simulink model "DoublePendSim"  (R2022b)
settings: Solver=ode1be  StartTime=0.0  StopTime=3  FixedStep=0.01  RelTol=1e-3
model workspace (MAT data in the model file):
  E = Simulink.Parameter
  E.Value = [1; 1; 0.5; 0; 0.5; 0]
  E.DataType = 'auto'
  E.Complexity = 'real'
  E.Dimensions = [6 1]
  F = Simulink.Parameter
  F.Value = [-1137.64638281  0.333333333333  284.601832874  -0.333333333333  -32.6215233406  -0.333333333333; 1935122.34305  -0.666666666667  -1227588.90432  -0.333333333333  -1810907.99136  -0.333333333333; 314.687310794  -0.333333333333  -490.937143366  0.833333333333  -190.967975417  -0.166666666667; 1036610.18685  0  -658628.221442  0  -949391.226529  0; -27.639193223  -0.333333333333  -190.739049358  -0.166666666667  -1000.74980716  0.833333333333; 1028988.90962  0  -652879.570619  0  -976734.231834  0]
  F.DataType = 'auto'
  F.Complexity = 'real'
  F.Dimensions = [6 6]
  H = Simulink.Parameter
  H.Value = [0.666666666667  0.333333333333  0.333333333333; 0.666666666667  0.333333333333  0.333333333333; 0.333333333333  0.166666666667  0.166666666667; 0  0  0; 0.333333333333  0.166666666667  0.166666666667; 0  0  0]
  H.DataType = 'auto'
  H.Complexity = 'real'
  H.Dimensions = [6 3]
  K1 = Simulink.Parameter
  K1.Value = [1137.64638281  -284.601832874  32.6215233406; -1935122.34305  1227578.3936  1810909.04243; -314.687310794  490.937143366  190.967975417; -1036610.18685  658699.6943  949372.307244; 27.639193223  190.739049358  1000.74980716; -1028988.90962  652728.216333  976843.543262]
  K1.DataType = 'auto'
  K1.Complexity = 'real'
  K1.Dimensions = [6 3]
  K2 = Simulink.Parameter
  K2.Value = [-674.215263137  -337.107631568  -337.107631568; 277248.819028  138624.409514  138624.409514; -17.7323879538  -8.8661939769  -8.8661939769; 155066.975241  77533.4876207  77533.4876207; -415.811303211  -207.905651605  -207.905651605; 142788.005598  71394.0027992  71394.0027992]
  K2.DataType = 'auto'
  K2.Complexity = 'real'
  K2.Dimensions = [6 3]
  T = Simulink.Parameter
  T.Value = [0.333333333333  0  -0.333333333333  0  -0.333333333333  0; -0.666666666667  1  -0.333333333333  0  -0.333333333333  0; -0.333333333333  0  0.833333333333  0  -0.166666666667  0; 0  0  0  1  0  0; -0.333333333333  0  -0.166666666667  0  0.833333333333  0; 0  0  0  0  0  1]
  T.DataType = 'auto'
  T.Complexity = 'real'
  T.Dimensions = [6 6]
values from neighbouring files (symbols this model uses):
  A = [A(1,:);A(4,:);A(2,:);A(5,:);A(3,:);A(6,:)]    [DoublePendCart.m]
  B = [B(1);B(4);B(2);B(5);B(3);B(6)]    [DoublePendCart.m]
  C = [1,zeros(1,5) ... (first row only)    [DoublePendCart.m]
  F = T*A-K1*C    [DoublePendCart.m]
  H = E*pinv(C*E)    [DoublePendCart.m]
  K1 = place((T*A)',C',10*[-8,-30,-2,-100,-3,-120])'    [DoublePendCart.m]
  K2 = F*H    [DoublePendCart.m]
  K_c = place(A,B,[-8,-30,-2,-100,-3,-120])    [DoublePendCart.m]
  L = place(A',C',10*[-8,-30,-2,-100,-3,-120])'    [DoublePendCart.m]
  T = eye(size(H*C,1))-H*C    [DoublePendCart.m]
settings Model: Creator=Razvan  LastModifiedBy=Razvan
settings SolverCC: MaxConsecutiveZCs=1  MaxConsecutiveMinStep=auto  ZeroCrossControl=EnableAll  ZeroCrossAlgorithm=Adaptive  SolverResetMethod=Robust  DecoupledContinuousIntegration=on  MinimalZcImpactIntegration=on  ODENIntegrationMethod=ode5  MaxZcPerStep=100  MaxZcBracketingIterations=50
settings DebuggingCC: IgnoredZcDiagnostic=none

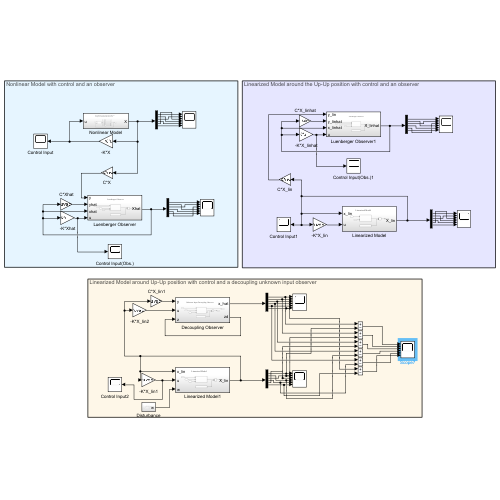
[thumbnail: Simulink's stored preview of the top-level diagram]
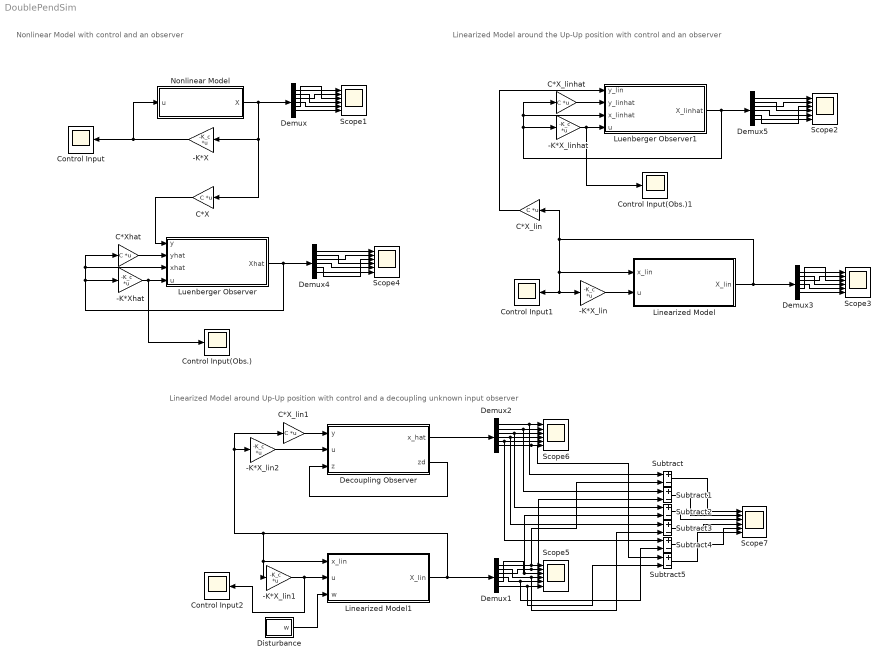
== system DoublePendSim ==
  note: Linearized Model around Up-Up position with control and a decoupling unknown input observer
  note: Linearized Model around the Up-Up position with control and an observer
  note: Nonlinear Model with control and an observer
  -K*X : Gain  Gain=-K_c  Multiplication=Matrix(K*u)
  -K*X_lin : Gain  Gain=-K_c  Multiplication=Matrix(K*u) (u vector)
  -K*X_lin1 : Gain  Gain=-K_c  Multiplication=Matrix(K*u) (u vector)
  -K*X_lin2 : Gain  Gain=-K_c  Multiplication=Matrix(K*u) (u vector)
  -K*X_linhat : Gain  Gain=-K_c  Multiplication=Matrix(K*u)
  -K*Xhat : Gain  Gain=-K_c  Multiplication=Matrix(K*u)
  C*X : Gain  Gain=C  Multiplication=Matrix(K*u) (u vector)
  C*X_lin : Gain  Gain=C  Multiplication=Matrix(K*u) (u vector)
  C*X_lin1 : Gain  Gain=C  Multiplication=Matrix(K*u) (u vector)
  C*X_linhat : Gain  Gain=C  Multiplication=Matrix(K*u) (u vector)
  C*Xhat : Gain  Gain=C  Multiplication=Matrix(K*u) (u vector)
  Control Input : Scope
  Control Input(Obs.) : Scope
  Control Input(Obs.)1 : Scope
  Control Input1 : Scope
  Control Input2 : Scope
  Decoupling Observer : Subsystem
  Demux{,1..5} (6 alike) : Demux  Outputs=6
  Disturbance : Subsystem
  Linearized Model : Subsystem
  Linearized Model1 : Subsystem
  Luenberger Observer : Subsystem
  Luenberger Observer1 : Subsystem
  Nonlinear Model : Subsystem
  Scope{1..7} (7 alike) : Scope  NumInputPorts=6
  Subtract{,1..5} (6 alike) : Sum  Inputs=+-
  wires:
  Nonlinear Model/1(X) -> Demux/1, C*X/1, -K*X/1
  -K*X/1 -> Nonlinear Model/1(u), Control Input/1
  Demux/1 -> Scope1/1
  Demux/3 -> Scope1/2
  Demux/5 -> Scope1/3
  Demux/2 -> Scope1/4
  Demux/4 -> Scope1/5
  Demux/6 -> Scope1/6
  -K*Xhat/1 -> Control Input(Obs.)/1, Luenberger Observer/4(u)
  C*Xhat/1 -> Luenberger Observer/2(yhat)
  C*X/1 -> Luenberger Observer/1(y)
  Demux4/2 -> Scope4/4
  Demux4/1 -> Scope4/1
  Demux4/3 -> Scope4/2
  Demux4/4 -> Scope4/5
  Demux4/5 -> Scope4/3
  Demux4/6 -> Scope4/6
  Luenberger Observer/1(Xhat) -> C*Xhat/1, Luenberger Observer/3(xhat), -K*Xhat/1, Demux4/1
  -K*X_lin/1 -> Linearized Model/2(u)
  Demux3/6 -> Scope3/6
  Demux3/4 -> Scope3/5
  Demux3/2 -> Scope3/4
  Demux3/5 -> Scope3/3
  Demux3/3 -> Scope3/2
  Demux3/1 -> Scope3/1
  Linearized Model/1(X_lin) -> Linearized Model/1(x_lin), Control Input1/1, -K*X_lin/1, C*X_lin/1, Demux3/1
  Luenberger Observer1/1(X_linhat) -> Demux5/1, -K*X_linhat/1, Luenberger Observer1/3(x_linhat), C*X_linhat/1
  Demux5/6 -> Scope2/6
  Demux5/5 -> Scope2/3
  Demux5/4 -> Scope2/5
  Demux5/3 -> Scope2/2
  Demux5/1 -> Scope2/1
  Demux5/2 -> Scope2/4
  C*X_lin/1 -> Luenberger Observer1/1(y_lin)
  C*X_linhat/1 -> Luenberger Observer1/2(y_linhat)
  -K*X_linhat/1 -> Luenberger Observer1/4(u), Control Input(Obs.)1/1
  -K*X_lin1/1 -> Linearized Model1/2(u), Control Input2/1
  Linearized Model1/1(X_lin) -> Demux1/1, C*X_lin1/1, -K*X_lin2/1, -K*X_lin1/1, Linearized Model1/1(x_lin)
  Demux1/1 -> Subtract/2, Scope5/1
  Demux1/3 -> Subtract1/2, Scope5/2
  Demux1/5 -> Scope5/3, Subtract2/2
  Demux1/2 -> Subtract3/2, Scope5/4
  Demux1/4 -> Subtract4/2, Scope5/5
  Demux1/6 -> Subtract5/2, Scope5/6
  Decoupling Observer/1(x_hat) -> Demux2/1
  Demux2/1 -> Subtract/1, Scope6/1
  Demux2/2 -> Subtract1/1, Scope6/2
  Demux2/3 -> Subtract2/1, Scope6/3
  Demux2/4 -> Subtract3/1, Scope6/4
  Demux2/5 -> Scope6/5, Subtract4/1
  Demux2/6 -> Subtract5/1, Scope6/6
  Decoupling Observer/2(zd) -> Decoupling Observer/3(z)
  -K*X_lin2/1 -> Decoupling Observer/2(u)
  C*X_lin1/1 -> Decoupling Observer/1(y)
  Subtract/1 -> Scope7/1
  Subtract1/1 -> Scope7/2
  Subtract2/1 -> Scope7/3
  Subtract3/1 -> Scope7/4
  Subtract4/1 -> Scope7/5
  Subtract5/1 -> Scope7/6
  Disturbance/1(w) -> Linearized Model1/3(w)

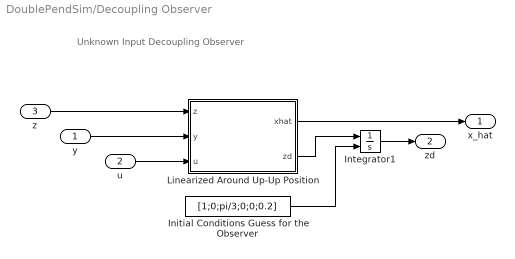
== system DoublePendSim/Decoupling Observer ==
  note: Unknown Input Decoupling Observer
  y : Inport
  u : Inport  Port=2
  z : Inport  Port=3
  Initial Conditions Guess for the Observer : Constant  Value=[1;0;pi/3;0;0;0.2]  VectorParams1D=off
  Integrator1 : Integrator  InitialConditionSource=external  InitialCondition=[0;0;pi/15;0;0;0]
  Linearized Around Up-Up Position : MATLAB Function  TreatAsAtomicUnit=on
  x_hat : Outport
  zd : Outport  Port=2
  wires:
  y/1 -> Linearized Around Up-Up Position/2(y)
  Linearized Around Up-Up Position/1(xhat) -> x_hat/1
  u/1 -> Linearized Around Up-Up Position/3(u)
  z/1 -> Linearized Around Up-Up Position/1(z)
  Integrator1/1 -> zd/1
  Initial Conditions Guess for the Observer/1 -> Integrator1/2
  Linearized Around Up-Up Position/2(zd) -> Integrator1/1

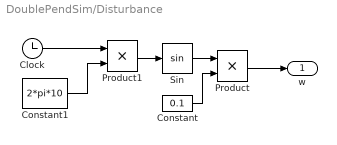
== system DoublePendSim/Disturbance ==
  Clock : Clock
  Constant : Constant  Value=0.1
  Constant1 : Constant  Value=2*pi*10
  Product : Product
  Product1 : Product
  Sin : Trigonometry
  w : Outport
  wires:
  Constant1/1 -> Product1/2
  Clock/1 -> Product1/1
  Product1/1 -> Sin/1
  Constant/1 -> Product/2
  Sin/1 -> Product/1
  Product/1 -> w/1

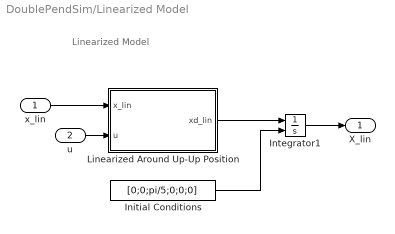
== system DoublePendSim/Linearized Model ==
  note: Linearized Model
  x_lin : Inport
  u : Inport  Port=2
  Initial Conditions : Constant  Value=[0;0;pi/5;0;0;0]  VectorParams1D=off
  Integrator1 : Integrator  InitialConditionSource=external  InitialCondition=[0;0;pi/15;0;0;0]
  Linearized Around Up-Up Position : MATLAB Function  TreatAsAtomicUnit=on
  X_lin : Outport
  wires:
  Initial Conditions/1 -> Integrator1/2
  Integrator1/1 -> X_lin/1
  u/1 -> Linearized Around Up-Up Position/2(u)
  x_lin/1 -> Linearized Around Up-Up Position/1(x_lin)
  Linearized Around Up-Up Position/1(xd_lin) -> Integrator1/1

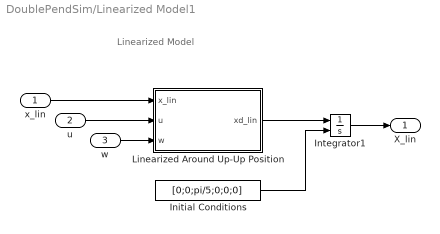
== system DoublePendSim/Linearized Model1 ==
  note: Linearized Model
  x_lin : Inport
  u : Inport  Port=2
  w : Inport  Port=3
  Initial Conditions : Constant  Value=[0;0;pi/5;0;0;0]  VectorParams1D=off
  Integrator1 : Integrator  InitialConditionSource=external  InitialCondition=[0;0;pi/15;0;0;0]
  Linearized Around Up-Up Position : MATLAB Function  TreatAsAtomicUnit=on
  X_lin : Outport
  wires:
  Linearized Around Up-Up Position/1(xd_lin) -> Integrator1/1
  x_lin/1 -> Linearized Around Up-Up Position/1(x_lin)
  u/1 -> Linearized Around Up-Up Position/2(u)
  Integrator1/1 -> X_lin/1
  Initial Conditions/1 -> Integrator1/2
  w/1 -> Linearized Around Up-Up Position/3(w)

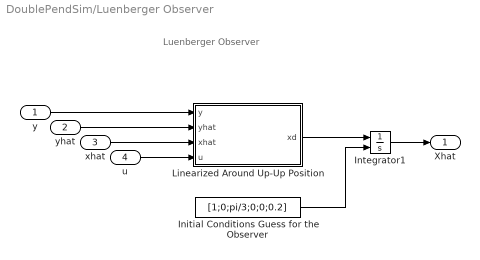
== system DoublePendSim/Luenberger Observer ==
  note: Luenberger Observer
  y : Inport
  yhat : Inport  Port=2
  xhat : Inport  Port=3
  u : Inport  Port=4
  Initial Conditions Guess for the Observer : Constant  Value=[1;0;pi/3;0;0;0.2]  VectorParams1D=off
  Integrator1 : Integrator  InitialConditionSource=external  InitialCondition=[0;0;pi/15;0;0;0]
  Linearized Around Up-Up Position : MATLAB Function  TreatAsAtomicUnit=on
  Xhat : Outport
  wires:
  yhat/1 -> Linearized Around Up-Up Position/2(yhat)
  Linearized Around Up-Up Position/1(xd) -> Integrator1/1
  xhat/1 -> Linearized Around Up-Up Position/3(xhat)
  u/1 -> Linearized Around Up-Up Position/4(u)
  y/1 -> Linearized Around Up-Up Position/1(y)
  Integrator1/1 -> Xhat/1
  Initial Conditions Guess for the Observer/1 -> Integrator1/2

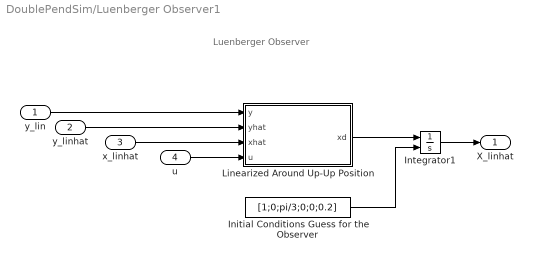
== system DoublePendSim/Luenberger Observer1 ==
  note: Luenberger Observer
  y_lin : Inport
  y_linhat : Inport  Port=2
  x_linhat : Inport  Port=3
  u : Inport  Port=4
  Initial Conditions Guess for the Observer : Constant  Value=[1;0;pi/3;0;0;0.2]  VectorParams1D=off
  Integrator1 : Integrator  InitialConditionSource=external  InitialCondition=[0;0;pi/15;0;0;0]
  Linearized Around Up-Up Position : MATLAB Function  TreatAsAtomicUnit=on
  X_linhat : Outport
  wires:
  Initial Conditions Guess for the Observer/1 -> Integrator1/2
  Integrator1/1 -> X_linhat/1
  y_lin/1 -> Linearized Around Up-Up Position/1(y)
  u/1 -> Linearized Around Up-Up Position/4(u)
  x_linhat/1 -> Linearized Around Up-Up Position/3(xhat)
  Linearized Around Up-Up Position/1(xd) -> Integrator1/1
  y_linhat/1 -> Linearized Around Up-Up Position/2(yhat)

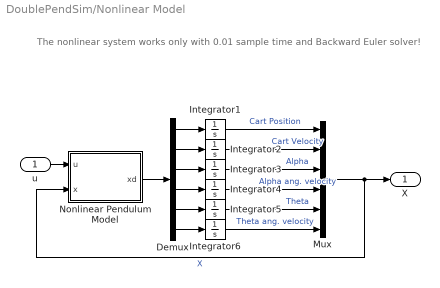
== system DoublePendSim/Nonlinear Model ==
  note: The nonlinear system works only with 0.01 sample time and Backward Euler solver!
  u : Inport
  Demux : Demux  Outputs=6
  Integrator1 : Integrator  ContinuousStateAttributes="\"Cart_Position\""
  Integrator2 : Integrator  ContinuousStateAttributes="\"Cart_Velocity\""
  Integrator3 : Integrator  InitialCondition=pi/10  WrapState=on  ContinuousStateAttributes="[\"Alpha_angle\"]"
  Integrator4 : Integrator  ContinuousStateAttributes="[\"Alpha_angular_velocity\"]"
  Integrator5 : Integrator  InitialCondition=pi/10  WrapState=on  ContinuousStateAttributes="[\"Theta_angle\"]"
  Integrator6 : Integrator  ContinuousStateAttributes="[\"Theta_angular_velocity\"]"
  Mux : Mux  Inputs=6
  Nonlinear Pendulum Model : MATLAB Function  TreatAsAtomicUnit=on
  X : Outport  Tag=da
  wires:
  Demux/3 -> Integrator3/1
  Nonlinear Pendulum Model/1(xd) -> Demux/1
  Demux/4 -> Integrator4/1
  Demux/1 -> Integrator1/1
  Integrator5/1 -> Mux/5  "Theta"
  Demux/5 -> Integrator5/1
  Integrator2/1 -> Mux/2  "Cart Velocity"
  Integrator6/1 -> Mux/6  "Theta ang. velocity"
  Demux/2 -> Integrator2/1
  Demux/6 -> Integrator6/1
  Integrator1/1 -> Mux/1  "Cart Position"
  Integrator4/1 -> Mux/4  "Alpha ang. velocity"
  Integrator3/1 -> Mux/3  "Alpha"
  u/1 -> Nonlinear Pendulum Model/1(u)
  Mux/1 -> X/1, Nonlinear Pendulum Model/2(x)  "X"

== matlab function DoublePendSim/Nonlinear Model/Nonlinear Pendulum Model ==
  data: u input size=1; x input size=6; xd output size=6
function xd = fcn(u,x)
xc = x(1); xcd = x(2); alpha = x(3); alphad = x(4); theta = x(5); thetad = x(6);
mc = 1; m1 = 1; m2 = 0.5;
l1 = 0.5; l2 = 0.25; g = 9.81;
a1 = mc+m1+m2; a2 = l1*(m1/2+m2);a3 = m2*l2/2; a4 = l1^2*(m1/3+m2); a5 = m2*l1*l2/2; a6 = m2*l2^2/3;
zeta1 = l1*g*(m1/2+m2); zeta2 = m2*l2*g/2;
xd = zeros(6,1);
xd(1) = xcd;
xd(2) = (zeta1*sin(alpha)*(a2*a6*cos(alpha) - a3*a5*cos(theta)*cos(alpha - theta)))/(a2^2*a6*cos(alpha)^2 - a1*a4*a6 + a3^2*a4*cos(theta)^2 + a1*a5^2*cos(alpha - theta)^2 - 2*a2*a3*a5*cos(alpha)*cos(theta)*cos(alpha - theta)) - thetad*((a5*thetad*sin(alpha - theta)*(a2*a6*cos(alpha) - a3*a5*cos(theta)*cos(alpha - theta)))/(a2^2*a6*cos(alpha)^2 - a1*a4*a6 + a3^2*a4*cos(theta)^2 + a1*a5^2*cos(alpha - theta)^2 - 2*a2*a3*a5*cos(alpha)*cos(theta)*cos(alpha - theta)) + (a3*thetad*sin(theta)*(a4*a6 - a5^2*cos(alpha - theta)^2))/(a2^2*a6*cos(alpha)^2 - a1*a4*a6 + a3^2*a4*cos(theta)^2 + a1*a5^2*cos(alpha - theta)^2 - 2*a2*a3*a5*cos(alpha)*cos(theta)*cos(alpha - theta))) - (u*(a4*a6 - a5^2*cos(alpha - theta)^2))/(a2^2*a6*cos(alpha)^2 - a1*a4*a6 + a3^2*a4*cos(theta)^2 + a1*a5^2*cos(alpha - theta)^2 - 2*a2*a3*a5*cos(alpha)*cos(theta)*cos(alpha - theta)) - alphad*((a2*alphad*sin(alpha)*(a4*a6 - a5^2*cos(alpha - theta)^2))/(a2^2*a6*cos(alpha)^2 - a1*a4*a6 + a3^2*a4*cos(theta)^2 + a1*a5^2*cos(alpha - theta)^2 - 2*a2*a3*a5*cos(alpha)*cos(theta)*cos(alpha - theta)) - (a5*alphad*sin(alpha - theta)*(a3*a4*cos(theta) - a2*a5*cos(alpha)*cos(alpha - theta)))/(a2^2*a6*cos(alpha)^2 - a1*a4*a6 + a3^2*a4*cos(theta)^2 + a1*a5^2*cos(alpha - theta)^2 - 2*a2*a3*a5*cos(alpha)*cos(theta)*cos(alpha - theta))) + (zeta2*sin(theta)*(a3*a4*cos(theta) - a2*a5*cos(alpha)*cos(alpha - theta)))/(a2^2*a6*cos(alpha)^2 - a1*a4*a6 + a3^2*a4*cos(theta)^2 + a1*a5^2*cos(alpha - theta)^2 - 2*a2*a3*a5*cos(alpha)*cos(theta)*cos(alpha - theta));
xd(3) = alphad;
xd(4) = thetad*((a5*thetad*sin(alpha - theta)*(a1*a6 - a3^2*cos(theta)^2))/(a2^2*a6*cos(alpha)^2 - a1*a4*a6 + a3^2*a4*cos(theta)^2 + a1*a5^2*cos(alpha - theta)^2 - 2*a2*a3*a5*cos(alpha)*cos(theta)*cos(alpha - theta)) + (a3*thetad*sin(theta)*(a2*a6*cos(alpha) - a3*a5*cos(theta)*cos(alpha - theta)))/(a2^2*a6*cos(alpha)^2 - a1*a4*a6 + a3^2*a4*cos(theta)^2 + a1*a5^2*cos(alpha - theta)^2 - 2*a2*a3*a5*cos(alpha)*cos(theta)*cos(alpha - theta))) + alphad*((a2*alphad*sin(alpha)*(a2*a6*cos(alpha) - a3*a5*cos(theta)*cos(alpha - theta)))/(a2^2*a6*cos(alpha)^2 - a1*a4*a6 + a3^2*a4*cos(theta)^2 + a1*a5^2*cos(alpha - theta)^2 - 2*a2*a3*a5*cos(alpha)*cos(theta)*cos(alpha - theta)) + (a5*alphad*sin(alpha - theta)*(a1*a5*cos(alpha - theta) - a2*a3*cos(alpha)*cos(theta)))/(a2^2*a6*cos(alpha)^2 - a1*a4*a6 + a3^2*a4*cos(theta)^2 + a1*a5^2*cos(alpha - theta)^2 - 2*a2*a3*a5*cos(alpha)*cos(theta)*cos(alpha - theta))) + (u*(a2*a6*cos(alpha) - a3*a5*cos(theta)*cos(alpha - theta)))/(a2^2*a6*cos(alpha)^2 - a1*a4*a6 + a3^2*a4*cos(theta)^2 + a1*a5^2*cos(alpha - theta)^2 - 2*a2*a3*a5*cos(alpha)*cos(theta)*cos(alpha - theta)) - (zeta1*sin(alpha)*(a1*a6 - a3^2*cos(theta)^2))/(a2^2*a6*cos(alpha)^2 - a1*a4*a6 + a3^2*a4*cos(theta)^2 + a1*a5^2*cos(alpha - theta)^2 - 2*a2*a3*a5*cos(alpha)*cos(theta)*cos(alpha - theta)) + (zeta2*sin(theta)*(a1*a5*cos(alpha - theta) - a2*a3*cos(alpha)*cos(theta)))/(a2^2*a6*cos(alpha)^2 - a1*a4*a6 + a3^2*a4*cos(theta)^2 + a1*a5^2*cos(alpha - theta)^2 - 2*a2*a3*a5*cos(alpha)*cos(theta)*cos(alpha - theta));
xd(5) = thetad;
xd(6) = (u*(a3*a4*cos(theta) - a2*a5*cos(alpha)*cos(alpha - theta)))/(a2^2*a6*cos(alpha)^2 - a1*a4*a6 + a3^2*a4*cos(theta)^2 + a1*a5^2*cos(alpha - theta)^2 - 2*a2*a3*a5*cos(alpha)*cos(theta)*cos(alpha - theta)) - alphad*((a5*alphad*sin(alpha - theta)*(a1*a4 - a2^2*cos(alpha)^2))/(a2^2*a6*cos(alpha)^2 - a1*a4*a6 + a3^2*a4*cos(theta)^2 + a1*a5^2*cos(alpha - theta)^2 - 2*a2*a3*a5*cos(alpha)*cos(theta)*cos(alpha - theta)) - (a2*alphad*sin(alpha)*(a3*a4*cos(theta) - a2*a5*cos(alpha)*cos(alpha - theta)))/(a2^2*a6*cos(alpha)^2 - a1*a4*a6 + a3^2*a4*cos(theta)^2 + a1*a5^2*cos(alpha - theta)^2 - 2*a2*a3*a5*cos(alpha)*cos(theta)*cos(alpha - theta))) - thetad*((a5*thetad*sin(alpha - theta)*(a1*a5*cos(alpha - theta) - a2*a3*cos(alpha)*cos(theta)))/(a2^2*a6*cos(alpha)^2 - a1*a4*a6 + a3^2*a4*cos(theta)^2 + a1*a5^2*cos(alpha - theta)^2 - 2*a2*a3*a5*cos(alpha)*cos(theta)*cos(alpha - theta)) - (a3*thetad*sin(theta)*(a3*a4*cos(theta) - a2*a5*cos(alpha)*cos(alpha - theta)))/(a2^2*a6*cos(alpha)^2 - a1*a4*a6 + a3^2*a4*cos(theta)^2 + a1*a5^2*cos(alpha - theta)^2 - 2*a2*a3*a5*cos(alpha)*cos(theta)*cos(alpha - theta))) - (zeta2*sin(theta)*(a1*a4 - a2^2*cos(alpha)^2))/(a2^2*a6*cos(alpha)^2 - a1*a4*a6 + a3^2*a4*cos(theta)^2 + a1*a5^2*cos(alpha - theta)^2 - 2*a2*a3*a5*cos(alpha)*cos(theta)*cos(alpha - theta)) + (zeta1*sin(alpha)*(a1*a5*cos(alpha - theta) - a2*a3*cos(alpha)*cos(theta)))/(a2^2*a6*cos(alpha)^2 - a1*a4*a6 + a3^2*a4*cos(theta)^2 + a1*a5^2*cos(alpha - theta)^2 - 2*a2*a3*a5*cos(alpha)*cos(theta)*cos(alpha - theta));

== matlab function DoublePendSim/Linearized Model1/Linearized Around Up-Up Position ==
  data: x_lin input; u input; w input; xd_lin output; A parameter; B parameter; E parameter
function xd_lin = fcn(x_lin,u,w, A, B, E)
xd_lin = A*x_lin+B*u+E*w;

== matlab function DoublePendSim/Decoupling Observer/Linearized Around Up-Up Position ==
  data: z input; y input; u input; xhat output; zd output; F parameter; H parameter; T parameter; K1 parameter; K2 parameter; B parameter
function [xhat,zd] = fcn(z,y,u, F, H, T, K1, K2, B)
zd = F*z+T*B*u+(K1+K2)*y;
xhat=z+H*y;

== matlab function DoublePendSim/Linearized Model/Linearized Around Up-Up Position ==
  data: x_lin input; u input; xd_lin output; A parameter; B parameter
function xd_lin = fcn(x_lin,u, A, B)
xd_lin = A*x_lin+B*u;

== matlab function DoublePendSim/Luenberger Observer/Linearized Around Up-Up Position ==
  data: y input; yhat input; xhat input; u input; xd output; A parameter; B parameter; L parameter
function xd = fcn(y,yhat,xhat,u, A, B, L)

xd = A*xhat+B*u+L*(y-yhat);

== matlab function DoublePendSim/Luenberger Observer1/Linearized Around Up-Up Position ==
  data: y input; yhat input; xhat input; u input; xd output; A parameter; B parameter; L parameter
function xd = fcn(y,yhat,xhat,u, A, B, L)

xd = A*xhat+B*u+L*(y-yhat);
